simulink model "astron_hw_test_au50_64k_8in"  (R2021a)
settings: Solver=VariableStepDiscrete  StartTime=0.0  StopTime=32000  RelTol=1e-3
undefined symbols (not defined in the file): d0, d1, d2, d3, d4, d5, d6, d7, FFT, sr, Wideband_FFT
libraries: xbsIndex_r4 x1247, casper_library_misc x6, xps_library x1
(part 2 of 26)

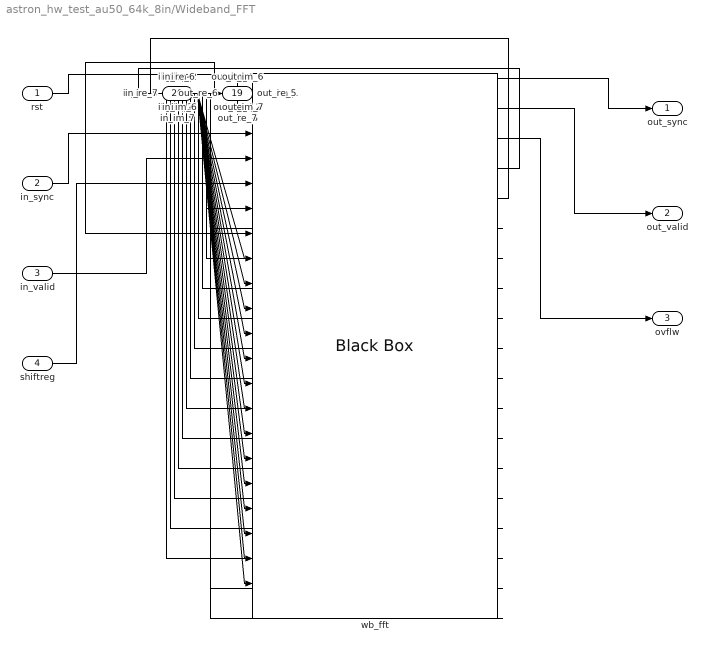
== system astron_hw_test_au50_64k_8in/Wideband_FFT ==
  rst : Inport
  in_sync : Inport  Port=2
  in_valid : Inport  Port=3
  shiftreg : Inport  Port=4
  in_im_0 : Inport  Port=5
  in_re_0 : Inport  Port=6
  in_im_1 : Inport  Port=7
  in_re_1 : Inport  Port=8
  in_im_2 : Inport  Port=9
  in_re_2 : Inport  Port=10
  in_im_3 : Inport  Port=11
  in_re_3 : Inport  Port=12
  in_im_4 : Inport  Port=13
  in_re_4 : Inport  Port=14
  in_im_5 : Inport  Port=15
  in_re_5 : Inport  Port=16
  in_im_6 : Inport  Port=17
  in_re_6 : Inport  Port=18
  in_im_7 : Inport  Port=19
  in_re_7 : Inport  Port=20
  wb_fft : xbsIndex_r4/Black Box  init_code=casper_wb_fft_config  sim_method=ISE Simulator  verbose=off  block_type=blackbox2
  out_sync : Outport  VectorParamsAs1DForOutWhenUnconnected=off
  out_valid : Outport  Port=2  VectorParamsAs1DForOutWhenUnconnected=off
  ovflw : Outport  Port=3  VectorParamsAs1DForOutWhenUnconnected=off
  out_im_0 : Outport  Port=4  VectorParamsAs1DForOutWhenUnconnected=off
  out_re_0 : Outport  Port=5  VectorParamsAs1DForOutWhenUnconnected=off
  out_im_1 : Outport  Port=6
  out_re_1 : Outport  Port=7
  out_im_2 : Outport  Port=8
  out_re_2 : Outport  Port=9
  out_im_3 : Outport  Port=10
  out_re_3 : Outport  Port=11
  out_im_4 : Outport  Port=12
  out_re_4 : Outport  Port=13
  out_im_5 : Outport  Port=14
  out_re_5 : Outport  Port=15
  out_im_6 : Outport  Port=16
  out_re_6 : Outport  Port=17
  out_im_7 : Outport  Port=18
  out_re_7 : Outport  Port=19
  wires:
  rst/1 -> wb_fft/1
  in_sync/1 -> wb_fft/2
  wb_fft/1 -> out_sync/1
  in_valid/1 -> wb_fft/3
  wb_fft/2 -> out_valid/1
  shiftreg/1 -> wb_fft/4
  wb_fft/3 -> ovflw/1
  in_im_0/1 -> wb_fft/5
  in_re_0/1 -> wb_fft/6
  wb_fft/4 -> out_im_0/1
  wb_fft/5 -> out_re_0/1
  in_im_1/1 -> wb_fft/7
  in_re_1/1 -> wb_fft/8
  wb_fft/6 -> out_im_1/1
  wb_fft/7 -> out_re_1/1
  in_im_2/1 -> wb_fft/9
  in_re_2/1 -> wb_fft/10
  wb_fft/8 -> out_im_2/1
  wb_fft/9 -> out_re_2/1
  in_im_3/1 -> wb_fft/11
  in_re_3/1 -> wb_fft/12
  wb_fft/10 -> out_im_3/1
  wb_fft/11 -> out_re_3/1
  in_im_4/1 -> wb_fft/13
  in_re_4/1 -> wb_fft/14
  wb_fft/12 -> out_im_4/1
  wb_fft/13 -> out_re_4/1
  in_im_5/1 -> wb_fft/15
  in_re_5/1 -> wb_fft/16
  wb_fft/14 -> out_im_5/1
  wb_fft/15 -> out_re_5/1
  in_im_6/1 -> wb_fft/17
  in_re_6/1 -> wb_fft/18
  wb_fft/16 -> out_im_6/1
  wb_fft/17 -> out_re_6/1
  in_im_7/1 -> wb_fft/19
  in_re_7/1 -> wb_fft/20
  wb_fft/18 -> out_im_7/1
  wb_fft/19 -> out_re_7/1
